simulink model "check_Powertrain"  (R2018b)
settings: configuration reference "Physics" (kept outside this file)
model workspace (MAT data in the model file):
  veh_param = Simulink.Parameter
  veh_param.Value.cLiftF = 0
  veh_param.Value.cLiftR = 0
  veh_param.Value.CoGx_m = 0
  veh_param.Value.CoGy_m = 0
  veh_param.Value.CoGz_m = 0
  veh_param.Value.cDrag = 0
  veh_param.Value.Aref_m2 = 0
  veh_param.Value.Gearratio = 0
  veh_param.Value.Wheelbase_m = 0
  veh_param.Value.PacLatF = [0 0 0 0 0]
  veh_param.Value.PacLongF = [0 0 0 0 0]
  veh_param.Value.PacLatR = [0 0 0 0 0]
  veh_param.Value.PacLongR = [0 0 0 0 0]
  veh_param.Value.cRollFriction_Npmps = 0
  veh_param.Value.MaxRollFriction_N = 0
  veh_param.Value.T_YawRate_s = 0
  veh_param.Value.T_LatVel_s = 0
  veh_param.Value.TrackWidthF_m = 0
  veh_param.Value.TrackWidthR_m = 0
  veh_param.Value.TireRadiusF_m = 0
  veh_param.Value.TireRadiusR_m = 0
  veh_param.Value.VehicleInertia_kgm2 = 0
  veh_param.Value.WheelInertiaF_kgm2 = 0
  veh_param.Value.WheelInertiaR_kgm2 = 0
  veh_param.Value.VehicleMass_kg = 0
  veh_param.Value.switchModelBlend_mps = 0
  veh_param.Value.PTLimitLowVel_N = 0
  veh_param.Value.switchModelVel_mps = 0
  veh_param.Value.T_Tire_s = 0
  veh_param.DataType = 'struct'
  veh_param.Dimensions = [1 1]
  x0_positionstates = Simulink.Parameter
  x0_positionstates.Value = [0 0 0]
  x0_positionstates.DataType = 'auto'
  x0_positionstates.Dimensions = [1 3]
settings Model: DataDictionary=vehicleparameters_vehdynsim.sldd  OrderedModelArguments=off  Creator=wischnewski  LastModifiedBy=ga25xiw

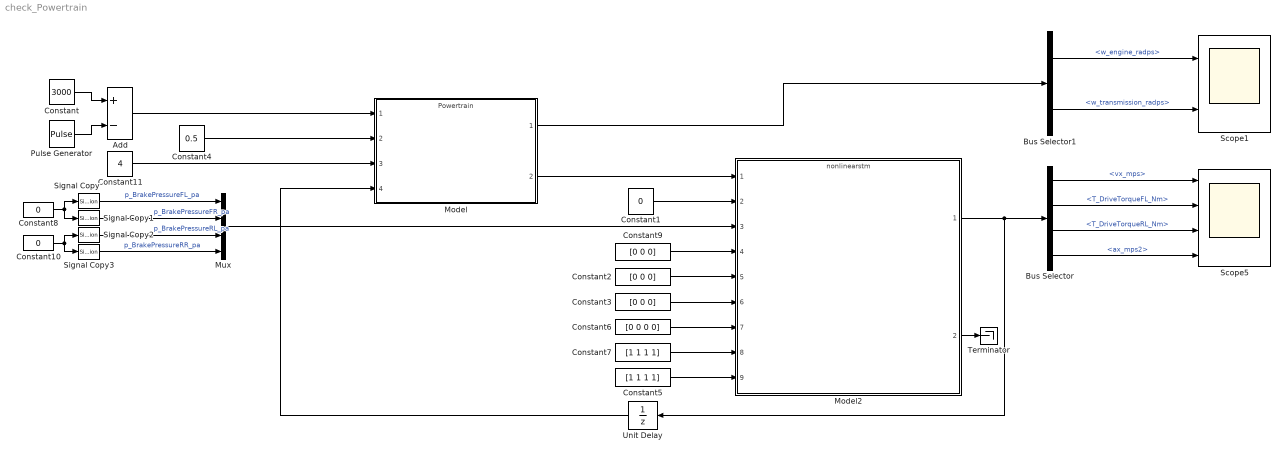
== system check_Powertrain ==
  Add : Sum  Inputs=+-
  Bus Selector : BusSelector  OutputSignals=vx_mps,T_DriveTorqueFL_Nm,T_DriveTorqueRL_Nm,ax_mps2
  Bus Selector1 : BusSelector  OutputSignals=w_engine_radps,w_transmission_radps
  Constant : Constant  Value=3000
  Constant1 : Constant  Value=0
  Constant10 : Constant  Value=0
  Constant11 : Constant  Value=4
  Constant2 : Constant  Value=[0 0 0]
  Constant3 : Constant  Value=[0 0 0]
  Constant4 : Constant  Value=0.5
  Constant5 : Constant  Value=[1 1 1 1]
  Constant6 : Constant  Value=[0 0 0 0]
  Constant7 : Constant  Value=[1 1 1 1]
  Constant8 : Constant  Value=0
  Constant9 : Constant  Value=[0 0 0]
  Model : ModelReference  ModelNameDialog=Powertrain.slx  SimulationMode=Normal  ModelReferenceVersion=1.915
  Model2 : ModelReference  ModelNameDialog=nonlinearstm  ParameterArgumentNames=x0_positionstates  ParameterArgumentValues=[0,0,0]  UsingDefaultArgumentValue=0  SimulationMode=Normal  ModelReferenceVersion=1.404
  Mux : Mux
  Pulse Generator : DiscretePulseGenerator  PulseType=Time based  Amplitude=3000  Period=150  PulseWidth=90  PhaseDelay=60
  Scope1 : Scope  NumInputPorts=2
  Scope5 : Scope  NumInputPorts=4
  Signal Copy{,1..3} (4 alike) : SignalConversion  OverrideOpt=off
  Terminator : Terminator
  Unit Delay : UnitDelay  SampleTime=-1
  wires:
  Model2/2 -> Terminator/1
  Constant1/1 -> Model2/2
  Constant2/1 -> Model2/5
  Bus Selector/1 -> Scope5/1  "<vx_mps>"
  Constant9/1 -> Model2/4
  Constant5/1 -> Model2/9
  Signal Copy3/1 -> Mux/4  "p_BrakePressureRR_pa"
  Constant10/1 -> Signal Copy3/1, Signal Copy2/1
  Mux/1 -> Model2/3
  Signal Copy2/1 -> Mux/3  "p_BrakePressureRL_pa"
  Signal Copy1/1 -> Mux/2  "p_BrakePressureFR_pa"
  Constant7/1 -> Model2/8
  Constant3/1 -> Model2/6
  Constant6/1 -> Model2/7
  Bus Selector/2 -> Scope5/2  "<T_DriveTorqueFL_Nm>"
  Constant8/1 -> Signal Copy1/1, Signal Copy/1
  Bus Selector/4 -> Scope5/4  "<ax_mps2>"
  Signal Copy/1 -> Mux/1  "p_BrakePressureFL_pa"
  Bus Selector/3 -> Scope5/3  "<T_DriveTorqueRL_Nm>"
  Constant/1 -> Add/1
  Pulse Generator/1 -> Add/2
  Add/1 -> Model/1
  Constant4/1 -> Model/2
  Constant11/1 -> Model/3
  Model2/1 -> Unit Delay/1, Bus Selector/1
  Unit Delay/1 -> Model/4
  Bus Selector1/1 -> Scope1/1  "<w_engine_radps>"
  Bus Selector1/2 -> Scope1/2  "<w_transmission_radps>"
  Model/2 -> Model2/1
  Model/1 -> Bus Selector1/1
